simulink model "Simulink_Xss_Com_Restricao"  (Simulink 8.2)
settings: Solver=ode4  SolverMode=SingleTasking  StartTime=0.0  StopTime=300  FixedStep=0.01  RelTol=1e-3
InitFcn:
  | Main_Simulink_Xss_Com_Restricao;
values from neighbouring files (symbols this model uses):
  A1 = [   1   0.1 ... (first row only)    [Matrizes.m]    (also in MatrizesEspacoEstados.m)
  B1 = [0 ... (first row only)    [Matrizes.m]    (also in MatrizesEspacoEstados.m)
  C = eye(n)    [Matrizes.m]    (also in MatrizesEspacoEstados.m)
  D = 0*C(:,n)    [Matrizes.m]    (also in MatrizesEspacoEstados.m)
  T = 1    [VariaveisDiversas_Restricoes.m]
undefined symbols (not defined in the file or in its folder): xk0
undefined symbols (not defined in the file): A, B, H, Umax
settings Model: Creator=Kawakami  LastModifiedBy=Eduardo
settings DataIOCC: LimitDataPoints=off  SaveOutput=off  SaveTime=off  TimeSaveName=t  SignalLoggingName=sigsOut
settings OptimizationCC: BooleanDataType=off
settings DebuggingCC: SaveWithParameterizedLinksMsg=none  SignalResolutionControl=TryResolveAllWithWarning  SolverPrmCheckMsg=none  MultiTaskDSMMsg=warning  MultiTaskCondExecSysMsg=none
settings HardwareCC: TargetUnknown=on
settings RTWCC: IncludeERTFirstTime=on

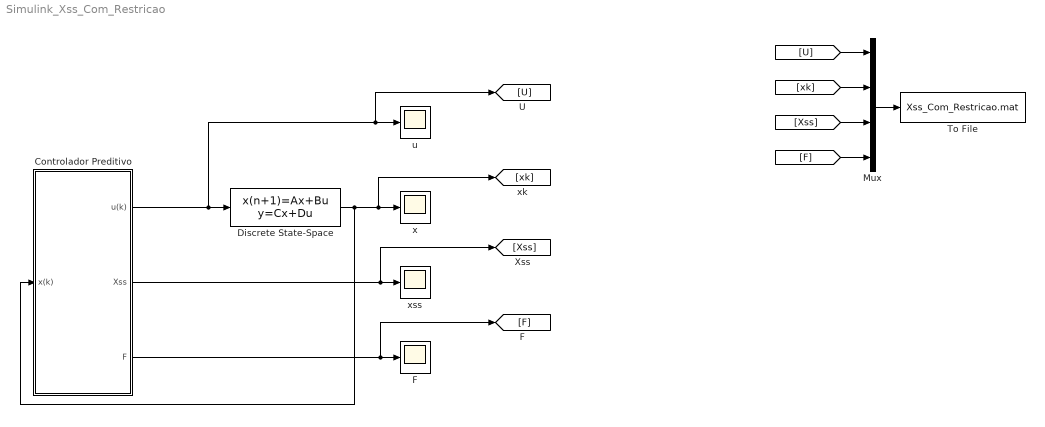
== system Simulink_Xss_Com_Restricao ==
  "Controlador Preditivo  " : Subsystem  mask{A=A, B=B, H=H, Umax=Umax, rho=0.00000001, T=T}
      mask prompts: A "Matriz Agregada A"; B "Matriz Agregada B"; H "Matriz H"; Umax "Restrição Entrada"; rho "Peso do Gamma"; T "T (passo da simulação)"
  Discrete State-Space : DiscreteStateSpace  A=A1  B=B1  C=C  D=D  X0=xk0  SampleTime=T
  F : Scope
      settings: YMin=-1.25  YMax=2.25  SaveName=ScopeData3
  Mux : Mux
  To File : ToFile  Filename=Xss_Com_Restricao.mat  MatrixName=XssComRestricao
  u : Scope
      settings: TimeRange=10  YMin=-2  YMax=0.5
  x : Scope
      settings: YMin=-1.25  YMax=2.25
  xss : Scope
      settings: YMin=-1.25  YMax=2.25  SaveName=ScopeData2
  wires:
  "Controlador Preditivo  "/1(u(k)) -> [U], u/1, Discrete State-Space/1
  Discrete State-Space/1 -> [xk], x/1, "Controlador Preditivo  "/1(x(k))
  "Controlador Preditivo  "/2(Xss) -> [Xss], xss/1
  "Controlador Preditivo  "/3(F) -> [F], F/1
  Mux/1 -> To File/1
  [xk] -> Mux/2
  [U] -> Mux/1
  [F] -> Mux/4
  [Xss] -> Mux/3

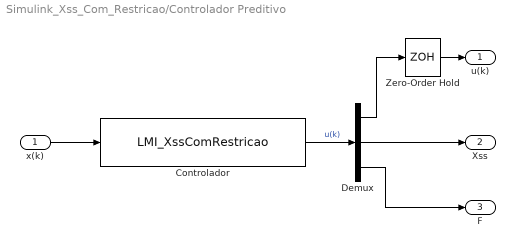
== system Simulink_Xss_Com_Restricao/Controlador Preditivo   ==
  x(k) : Inport
  Controlador : S-Function  FunctionName=LMI_XssComRestricao  Parameters=A, B, H, Umax, rho, T  EnableBusSupport=off
  Demux : Demux  Outputs=3
  Zero-Order Hold : ZeroOrderHold  SampleTime=T
  u(k) : Outport
  Xss : Outport  Port=2
  F : Outport  Port=3
  wires:
  Zero-Order Hold/1 -> u(k)/1
  x(k)/1 -> Controlador/1
  Controlador/1 -> Demux/1  "u(k)"
  Demux/1 -> Zero-Order Hold/1
  Demux/2 -> Xss/1
  Demux/3 -> F/1
